simulink model "sfcndemo_sfun_dynsize"  (Simulink 6.0)
settings: Solver=FixedStepDiscrete  StartTime=0.0  StopTime=10.0  RelTol=1e-3  AbsTol=1e-6
settings Model: Creator=The MathWorks Inc.  LastModifiedBy=batserve  ExtModeTrigMode=oneshot  ExtModeArmWhenConnect=off  ExtModeAutoUpdateStatusClock=off
settings DataIOCC: LimitDataPoints=off
settings OptimizationCC: BooleanDataType=off
settings DebuggingCC: CheckExecutionContextPreStartOutputMsg=on  CheckExecutionContextRuntimeOutputMsg=on  SolverPrmCheckMsg=none  InheritedTsInSrcMsg=none
settings HardwareCC: TargetUnknown=on

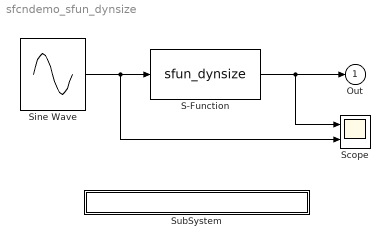
== system sfcndemo_sfun_dynsize ==
  S-Function : S-Function  FunctionName=sfun_dynsize
      mask Type: S-function: sfun_dynsize
      mask Display:
      | plot([1 NaN 2:6 NaN 19 NaN 1 NaN 2:6 NaN 19], [NaN 0 1 1 2 2 NaN 2 NaN NaN NaN 6 5 5 4 4 NaN 4  NaN]);
      | disp('Dynamic sized vector');
  Scope : Scope  NumInputPorts=2
      settings: YMin=-5~-5  YMax=5~5
  Sine Wave : Sin  Amplitude=1:4  SampleTime=0
  SubSystem : Subsystem  PropExecContextAcrossSSBoundary=on
      settings: OpenFcn=edit(fullfile(matlabroot,'simulink','src','sfun_dynsize.c'))
      mask Display: disp('matlabroot\simulink\src\sfun_dynsize.c');
  Out : Outport  InitialOutput=0
  wires:
  S-Function/1 -> Out/1, Scope/1
  Sine Wave/1 -> S-Function/1, Scope/2

== system sfcndemo_sfun_dynsize/SubSystem ==
